simulink model "oppg3d"  (R2024a)
settings: Solver=VariableStepAuto  StartTime=0.0  StopTime=10  RelTol=1e-3
values from neighbouring files (symbols this model uses):
  J = 15    [initverdier.m]
  k = 100    [initverdier.m]
  k_2 = 5    [initverdier.m]
  k_3 = 1    [initverdier.m]
  k_4 = 1    [initverdier.m]
  m = 200    [initverdier.m]
  theta_0 = 0    [initverdier.m]
settings Model: Creator=Lars André  LastModifiedBy=Lars André

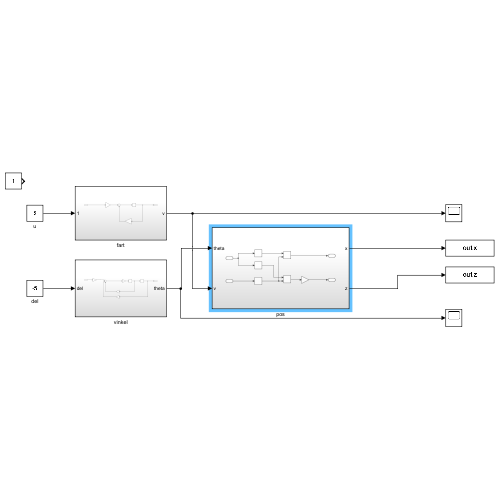
[thumbnail: Simulink's stored preview of the top-level diagram]
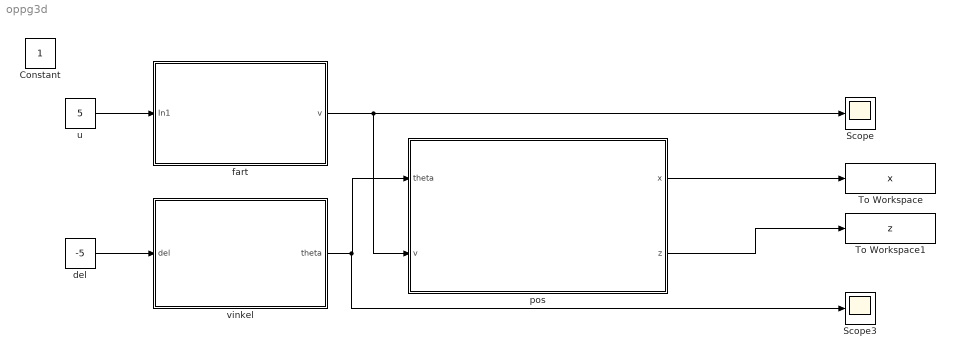
== system oppg3d ==
  Constant : Constant
  Scope : Scope
  Scope3 : Scope
  To Workspace : ToWorkspace  VariableName=x  SaveFormat=Timeseries  SampleTime=-1
  To Workspace1 : ToWorkspace  VariableName=z  SaveFormat=Timeseries  SampleTime=-1
  del : Constant  Value=-5
  fart : Subsystem
  pos : Subsystem
  u : Constant  Value=5
  vinkel : Subsystem
  wires:
  u/1 -> fart/1(In1)
  del/1 -> vinkel/1(del)
  fart/1(v) -> Scope/1, pos/2(v)
  vinkel/1(theta) -> Scope3/1, pos/1(theta)
  pos/1(x) -> To Workspace/1
  pos/2(z) -> To Workspace1/1

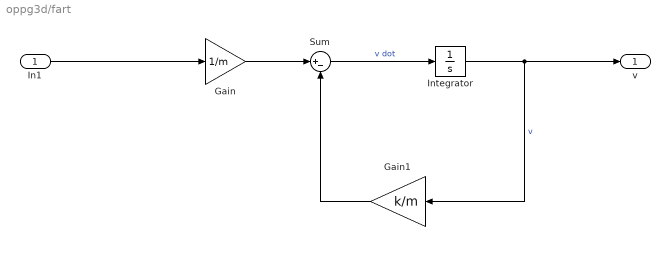
== system oppg3d/fart ==
  In1 : Inport
  Gain : Gain  Gain=1/m
  Gain1 : Gain  Gain=k/m
  Integrator : Integrator
  Sum : Sum  Inputs=|+-
  v : Outport
  wires:
  Integrator/1 -> v/1, Gain1/1  "v"
  In1/1 -> Gain/1
  Sum/1 -> Integrator/1  "v dot"
  Gain/1 -> Sum/1
  Gain1/1 -> Sum/2

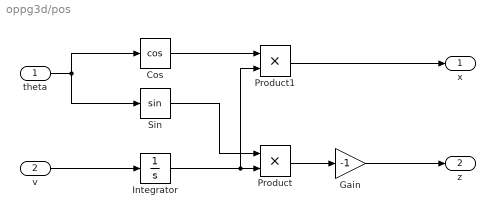
== system oppg3d/pos ==
  theta : Inport
  v : Inport  Port=2
  Cos : Trigonometry  Operator=cos
  Gain : Gain  Gain=-1
  Integrator : Integrator
  Product : Product
  Product1 : Product
  Sin : Trigonometry
  x : Outport
  z : Outport  Port=2
  wires:
  v/1 -> Integrator/1
  theta/1 -> Cos/1, Sin/1
  Integrator/1 -> Product1/2, Product/2
  Sin/1 -> Product/1
  Product/1 -> Gain/1
  Gain/1 -> z/1
  Cos/1 -> Product1/1
  Product1/1 -> x/1

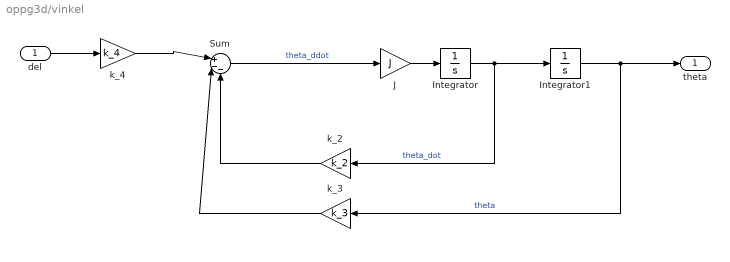
== system oppg3d/vinkel ==
  del : Inport
  Integrator : Integrator
  Integrator1 : Integrator  InitialCondition=theta_0
  J : Gain  Gain=J
  Sum : Sum  Inputs=|+--
  k_2 : Gain  Gain=k_2
  k_3 : Gain  Gain=k_3
  k_4 : Gain  Gain=k_4
  theta : Outport
  wires:
  Integrator/1 -> Integrator1/1, k_2/1  "theta_dot"
  Integrator1/1 -> theta/1, k_3/1  "theta"
  Sum/1 -> J/1  "theta_ddot"
  del/1 -> k_4/1
  k_4/1 -> Sum/1
  J/1 -> Integrator/1
  k_3/1 -> Sum/2
  k_2/1 -> Sum/3
